simulink library "intertravamento"  (R2015a)
settings: Solver=ode45  SolverMode=SingleTasking  StartTime=0.0  StopTime=10.0  RelTol=1e-3
PostLoadFcn:
  | setsysloc_simulink(bdroot)
undefined symbols (not defined in the file or in its folder): docblock, getdatatypespecs, NumBits1, NumBits2, sfunxy, sigbuilder_block, slcm, SlDemoSign, Slope1, Slope2
libraries: simulink x46, sl_helperblocks x2, eml_lib x1
(part 5 of 6)

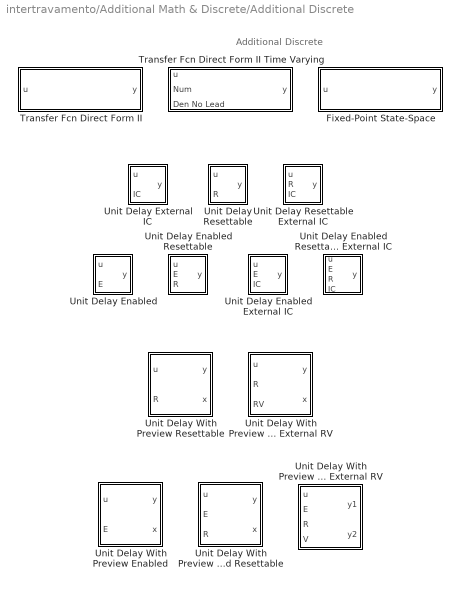
== system intertravamento/Additional Math & Discrete/Additional Discrete ==
  note: Additional Discrete
  Fixed-Point State-Space : Subsystem  mask(Fixed-Point State-Space){A=[2.6020 -2.2793 0.6708; 1 0 0; 0 1 0], B=[ 1; 0; 0], C=[0.0184    0.0024    0.0055], D=[0.0033], X0=0.0, InternalDataType=fixdt('double'), StateEqScaling=2^0, OutputEqScaling=2^0, LockScale=off, RndMeth=Floor, DoSatur=off}
      mask prompts: A "Simulink:masks:StateMatrixA_MP"; B "Simulink:masks:InputMatrixB_MP"; C "Simulink:masks:OutputMatrixC_MP"; D "Simulink:masks:DirectFeedthroughMatrixD_MP"; X0 "Simulink:masks:InitialConditionForState_MP"; InternalDataType "Simulink:masks:DataTypeForInternalCalculations_MP"; StateEqScaling "Simulink:masks:ScalingForStateEquationAXBU_MP"; OutputEqScaling "Simulink:masks:ScalingForOutputEquationCXDU_MP"; LockScale "Simulink:masks:LockOutputDataTypeAgainstFxpTools_MP"; RndMeth "Simulink:masks:IntegerRoundingMode_MP"; DoSatur "Simulink:masks:SaturateToMaxOrMinWhenOverflowsOccur_MP"
      mask help: Simulink:masks:FixedPointStateSpace_MD
      mask init:
      | blkH = gcbh;
      | blkName = getfullname(blkH);
      | 
      | vRndMeth = get_param(blkH,'RndMeth');
      | vDoSatur = get_param(blkH,'DoSatur');
      | blks = {'State Matrix A','Input Matrix B','Output Matrix C','Direct Link Matrix D','Sum Output Equation','Sum State Equation','Downcast Next State X','Downcast Output Y'};
      | for i = 1:length(blks)
      |   set_param([blkName,'/',blks{i}],'RndMeth',vRndMeth, ...
      | 	  'DoSatur',vDoSatur);
      | end
      mask TypeOptions RndMeth: Simulink:masks:Ceiling | Simulink:masks:Convergent | Simulink:masks:Floor | Simulink:masks:Nearest | Simulink:masks:Round | Simulink:masks:Simplest | Simulink:masks:Zero
      mask Display:
      | text(0.5, 0.5, 'y(n)=Cx(n)+Du(n)', 'horizontalAlignment', 'center', 'verticalAlignment', 'bottom');
      | text(0.5, 0.5, 'x(n+1)=Ax(n)+Bu(n)', 'horizontalAlignment', 'center', 'verticalAlignment', 'top');
  Transfer Fcn Direct Form II : Subsystem  mask(Transfer Fcn Direct Form II){NumCoefVec=[0.2 0.3 0.2], DenCoefVec=[-0.9    0.6], vinit=0.0, RndMeth=Floor, DoSatur=off}
      mask prompts: NumCoefVec "Simulink:masks:NumeratorCoefficients_MP"; DenCoefVec "Simulink:masks:DenominatorCoefficientsExcludingLead_MP"; vinit "Simulink:masks:InitialCondition_MP"; RndMeth "Simulink:masks:IntegerRoundingMode_MP"; DoSatur "Simulink:masks:SaturateToMaxOrMinWhenOverflowsOccur_MP"
      mask help: Simulink:masks:TransferFcnDirectFormII_MD
      mask init:
      | blkH = gcbh;
      | blkName = getfullname(blkH);
      | 
      | vRndMeth = get_param(blkH,'RndMeth');
      | vDoSatur = get_param(blkH,'DoSatur');
      | DCGain = polyval(NumCoefVec,1)./polyval([1 DenCoefVec],1);
      | maxGain = max( 1, max(max(abs(DCGain))) );
      | maxGain = max( maxGain, abs(NumCoefVec(1)) );
      | OutputSlopeMult = double(2^ceil(log2(maxGain)));
      | DCGain = (1)./polyval([1 DenCoefVec],1);
      | maxGain = max( 1, max(max(abs(DCGain))) );
      | OutputSlopeMult2 = double(2^ceil(log2(maxGain)));
      | set_param([blkName,'/NumCoef'],'RndMeth',vRndMeth, ...
      | 	'DoSatur',vDoSatur);
      | set_param([blkName,'/DenCoef'],'RndMeth',vRndMeth, ...
      | 	'DoSatur',vDoSatur);
      | set_param([blkName,'/Downcast'],'RndMeth',vRndMeth, ...
      | 	'DoSatur',vDoSatur);
      | set_param([blkName,'/Downcast1'],'RndMeth',vRndMeth, ...
      | 	'DoSatur',vDoSatur);
      | set_param([blkName,'/Sum'],'RndMeth',vRndMeth, ...
      | 	'DoSatur',vDoSatur);
      mask TypeOptions RndMeth: Simulink:masks:Ceiling | Simulink:masks:Convergent | Simulink:masks:Floor | Simulink:masks:Nearest | Simulink:masks:Round | Simulink:masks:Simplest | Simulink:masks:Zero
      mask Display: dpoly(NumCoefVec,[1 DenCoefVec],'z-')
  Transfer Fcn Direct Form II Time Varying : Subsystem  mask(Transfer Fcn Direct Form II Time Varying){vinit=0.0, RndMeth=Floor, DoSatur=off}
      mask prompts: vinit "Simulink:masks:InitialCondition_MP"; RndMeth "Simulink:masks:IntegerRoundingMode_MP"; DoSatur "Simulink:masks:SaturateToMaxOrMinWhenOverflowsOccur_MP"
      mask help: Simulink:masks:TransferFcnDirectFormIITimeVarying_MD
      mask init:
      | blkH = gcbh;
      | blkName = getfullname(blkH);
      | 
      | vRndMeth = get_param(blkH,'RndMeth');
      | vDoSatur = get_param(blkH,'DoSatur');
      | set_param([blkName,'/Dot1'],'RndMeth',vRndMeth, ...
      | 	'DoSatur',vDoSatur);
      | set_param([blkName,'/Dot2'],'RndMeth',vRndMeth, ...
      | 	'DoSatur',vDoSatur);
      | set_param([blkName,'/Downcast'],'RndMeth',vRndMeth, ...
      | 	'DoSatur',vDoSatur);
      | set_param([blkName,'/Downcast1'],'RndMeth',vRndMeth, ...
      | 	'DoSatur',vDoSatur);
      | set_param([blkName,'/Sum'],'RndMeth',vRndMeth, ...
      | 	'DoSatur',vDoSatur);
      mask TypeOptions RndMeth: Simulink:masks:Ceiling | Simulink:masks:Convergent | Simulink:masks:Floor | Simulink:masks:Nearest | Simulink:masks:Round | Simulink:masks:Simplest | Simulink:masks:Zero
      mask Display: fprintf('Direct\nForm II')
  Unit Delay Enabled : Subsystem  mask(Unit Delay Enabled){vinit=0.0, tsamp=-1}
      mask prompts: vinit "Simulink:masks:InitialCondition_MP"; tsamp "Simulink:masks:SampleTime_MP"
      mask help: Simulink:masks:UnitDelayEnabled_MD
      mask Display: dpoly(1,[1 0],'z')
  Unit Delay Enabled External IC : Subsystem  mask(Unit Delay Enabled External Initial Condition){tsamp=-1}
      mask prompts: tsamp "Simulink:masks:SampleTime_MP"
      mask help: Simulink:masks:UnitDelayEnabledExternalInitialCondition_MD
      mask Display: dpoly(1,[1 0],'z')
  Unit Delay Enabled Resettable : Subsystem  mask(Unit Delay Enabled Resettable){vinit=0.0, tsamp=-1}
      mask prompts: vinit "Simulink:masks:InitialCondition_MP"; tsamp "Simulink:masks:SampleTime_MP"
      mask help: Simulink:masks:UnitDelayEnabledResettable_MD
      mask Display: dpoly(1,[1 0],'z')
  Unit Delay Enabled Resettable External IC : Subsystem  mask(Unit Delay Enabled Resettable External Initial Condition){tsamp=-1}
      mask prompts: tsamp "Simulink:masks:SampleTime_MP"
      mask help: Simulink:masks:UnitDelayEnabledResettableExternalInitialCondition_MD
      mask Display: dpoly(1,[1 0],'z')
  Unit Delay External IC : Subsystem  mask(Unit Delay External Initial Condition){tsamp=-1}
      mask prompts: tsamp "Simulink:masks:SampleTime_MP"
      mask help: Simulink:masks:UnitDelayExternalInitialCondition_MD
      mask Display: dpoly(1,[1 0],'z')
  Unit Delay Resettable : Subsystem  mask(Unit Delay Resettable){vinit=0.0, tsamp=-1}
      mask prompts: vinit "Simulink:masks:InitialCondition_MP"; tsamp "Simulink:masks:SampleTime_MP"
      mask help: Simulink:masks:UnitDelayResettable_MD
      mask Display: dpoly(1,[1 0],'z')
  Unit Delay Resettable External IC : Subsystem  mask(Unit Delay Resettable External Initial Condition){tsamp=-1}
      mask prompts: tsamp "Simulink:masks:SampleTime_MP"
      mask help: Simulink:masks:UnitDelayResettableExternalInitialCondition_MD
      mask Display: dpoly(1,[1 0],'z')
  Unit Delay With Preview Enabled : Subsystem  mask(Unit Delay With Preview Enabled){vinit=0.0, tsamp=-1}
      mask prompts: vinit "Simulink:masks:InitialCondition_MP"; tsamp "Simulink:masks:SampleTime_MP"
      mask help: Simulink:masks:UnitDelayWithPreviewEnabled_MD
      mask Display:
      | plot([NaN 0.1 0.13 0.1 NaN 0.1 0.13 0.1 NaN 0.1 0.13 0.1 NaN -0.05 0.025 0.075 0.13 NaN -0.05 0.025 0.075 0.13 NaN 0.13 0.13 0.4475 0.4475 0.13 NaN 0.4475 0.4975 0.5525 0.5225 0.5525 0.5225 NaN 0.4475 0.4975 1.05 NaN 0.5525 0.5525 0.87 0.87 0.5525 NaN 0.71125 0.71125 NaN 0.6525 0.77 NaN 0.6525 0.77 0.6525 0.77 NaN 0.87 0.92 1.05 NaN 0.92 0.92 0.075 0.075 0.13],[NaN 0.846666666666667 0.816666666666667 0.786666666666667 NaN 0.58 0.55 0.52 NaN 0.313333333333333 0.283333333333333 0.253333333333333 NaN 0.75 0.75 0.816666666666667 0.816666666666667 NaN 0.25 0.25 0.55 0.55 NaN 0.15 0.95 0.95 0.15 0.15 NaN 0.55 0.35 0.35 0.38 0.35 0.32 NaN 0.55 0.75 0.75 NaN 0.15 0.55 0.55 0.15 0.15 NaN 0.5 0.4 NaN 0.35 0.35 NaN 0.3 0.3 0.2 0.2 NaN 0.35 0.25 0.25 NaN 0.25 0.05 0.05 0.283333333333333 0.283333333333333]);
      | text(0.23,0.806666666666667,'u');
      | text(0.23,0.54,'E');
  Unit Delay With Preview Enabled Resettable : Subsystem  mask(Unit Delay With Preview Enabled Resettable){vinit=0.0, tsamp=-1}
      mask prompts: vinit "Simulink:masks:InitialCondition_MP"; tsamp "Simulink:masks:SampleTime_MP"
      mask help: Simulink:masks:UnitDelayWithPreviewEnabledResettable_MD
      mask Display:
      | plot([NaN 0.1 0.13 0.1 NaN 0.1 0.13 0.1 NaN 0.1 0.13 0.1 NaN 0.1 0.13 0.1 NaN -0.05 0.025 0.075 0.13 NaN -0.05 0.025 0.075 0.13 NaN -0.05 0.025 0.075 0.13 NaN 0.13 0.13 0.4475 0.4475 0.13 NaN 0.4475 0.4975 0.5525 0.5225 0.5525 0.5225 NaN 0.4475 0.4975 1.05 NaN 0.5525 0.5525 0.87 0.87 0.5525 NaN 0.71125 0.71125 NaN 0.6525 0.77 NaN 0.6525 0.77 0.6525 0.77 NaN 0.87 0.92 1.05 NaN 0.92 0.92 0.075 0.075 0.13],[NaN 0.88 0.85 0.82 NaN 0.68 0.65 0.62 NaN 0.48 0.45 0.42 NaN 0.28 0.25 0.22 NaN 0.833333333333333 0.833333333333333 0.85 0.85 NaN 0.5 0.5 0.65 0.65 NaN 0.166666666666667 0.166666666666667 0.45 0.45 NaN 0.15 0.95 0.95 0.15 0.15 NaN 0.55 0.35 0.35 0.38 0.35 0.32 NaN 0.55 0.75 0.75 NaN 0.15 0.55 0.55 0.15 0.15 NaN 0.5 0.4 NaN 0.35 0.35 NaN 0.3 0.3 0.2 0.2 NaN 0.35 0.25 0.25 NaN 0.25 0.05 0.05 0.25 0.25]);
      | text(0.23,0.84,'u');
      | text(0.23,0.64,'E');
      | text(0.23,0.44,'R');
  Unit Delay With Preview Enabled Resettable External RV : Subsystem  mask(Unit Delay With Preview Enabled Resettable External RV){vinit=0.0, tsamp=-1}
      mask prompts: vinit "Simulink:masks:InitialCondition_MP"; tsamp "Simulink:masks:SampleTime_MP"
      mask help: Simulink:masks:UnitDelayWithPreviewEnabledResettableExternalRV_MD
      mask Display:
      | plot([NaN 0.1 0.13 0.1 NaN 0.1 0.13 0.1 NaN 0.1 0.13 0.1 NaN 0.1 0.13 0.1 NaN 0.1 0.13 0.1 NaN -0.05 0.025 0.075 0.13 NaN -0.05 0.025 0.075 0.13 NaN -0.05 0.025 0.075 0.13 NaN -0.05 0.025 0.075 0.13 NaN 0.13 0.13 0.4475 0.4475 0.13 NaN 0.4475 0.4975 0.5525 0.5225 0.5525 0.5225 NaN 0.4475 0.4975 1.05 NaN 0.5525 0.5525 0.87 0.87 0.5525 NaN 0.71125 0.71125 NaN 0.6525 0.77 NaN 0.6525 0.77 0.6525 0.77 NaN 0.87 0.92 1.05 NaN 0.92 0.92 0.075 0.075 0.13],[NaN 0.9 0.87 0.84 NaN 0.74 0.71 0.68 NaN 0.58 0.55 0.52 NaN 0.42 0.39 0.36 NaN 0.26 0.23 0.2 NaN 0.875 0.875 0.87 0.87 NaN 0.625 0.625 0.71 0.71 NaN 0.375 0.375 0.55 0.55 NaN 0.125 0.125 0.39 0.39 NaN 0.15 0.95 0.95 0.15 0.15 NaN 0.55 0.35 0.35 0.38 0.35 0.32 NaN 0.55 0.75 0.75 NaN 0.15 0.55 0.55 0.15 0.15 NaN 0.5 0.4 NaN 0.35 0.35 NaN 0.3 0.3 0.2 0.2 NaN 0.35 0.25 0.25 NaN 0.25 0.05 0.05 0.23 0.23]);
      | text(0.23,0.86,'u');
      | text(0.23,0.7,'E');
      | text(0.23,0.54,'R');
      | text(0.23,0.38,'RV');
  Unit Delay With Preview Resettable : Subsystem  mask(Unit Delay With Preview Resettable){vinit=0.0, tsamp=-1}
      mask prompts: vinit "Simulink:masks:InitialCondition_MP"; tsamp "Simulink:masks:SampleTime_MP"
      mask help: Simulink:masks:UnitDelayWithPreviewResettable_MD
      mask Display:
      | plot([NaN 0.1 0.13 0.1 NaN 0.1 0.13 0.1 NaN -0.05 0.025 0.075 0.13 NaN -0.05 0.025 0.075 0.13 NaN 0.13 0.13 0.4475 0.4475 0.13 NaN 0.4475 0.4975 0.5525 0.5225 0.5525 0.5225 NaN 0.4475 0.4975 1.05 NaN 0.5525 0.5525 0.87 0.87 0.5525 NaN 0.71125 0.71125 NaN 0.6525 0.77 NaN 0.6525 0.77 0.6525 0.77 NaN 0.87 0.92 1.05],[NaN 0.755 0.725 0.695 NaN 0.305 0.275 0.245 NaN 0.75 0.75 0.725 0.725 NaN 0.25 0.25 0.275 0.275 NaN 0.0499999999999999 0.95 0.95 0.0499999999999999 0.0499999999999999 NaN 0.5 0.275 0.275 0.305 0.275 0.245 NaN 0.5 0.75 0.75 NaN 0.0499999999999999 0.5 0.5 0.0499999999999999 0.0499999999999999 NaN 0.45 0.325 NaN 0.275 0.275 NaN 0.225 0.225 0.0999999999999999 0.0999999999999999 NaN 0.275 0.25 0.25]);
      | text(0.23,0.715,'u');
      | text(0.23,0.265,'R');
  Unit Delay With Preview Resettable External RV : Subsystem  mask(Unit Delay With Preview Resettable External RV){vinit=0.0, tsamp=-1}
      mask prompts: vinit "Simulink:masks:InitialCondition_MP"; tsamp "Simulink:masks:SampleTime_MP"
      mask help: Simulink:masks:UnitDelayWithPreviewResettableExternalRV_MD
      mask Display:
      | plot([NaN 0.1 0.13 0.1 NaN 0.1 0.13 0.1 NaN 0.1 0.13 0.1 NaN -0.05 0.025 0.075 0.13 NaN -0.05 0.025 0.075 0.13 NaN -0.05 0.025 0.075 0.13 NaN 0.13 0.13 0.4475 0.4475 0.13 NaN 0.4475 0.4975 0.5525 0.5225 0.5525 0.5225 NaN 0.4475 0.4975 1.05 NaN 0.5525 0.5525 0.87 0.87 0.5525 NaN 0.71125 0.71125 NaN 0.6525 0.77 NaN 0.6525 0.77 0.6525 0.77 NaN 0.87 0.92 1.05],[NaN 0.83 0.8 0.77 NaN 0.53 0.5 0.47 NaN 0.23 0.2 0.17 NaN 0.833333333333333 0.833333333333333 0.8 0.8 NaN 0.5 0.5 0.5 0.5 NaN 0.166666666666667 0.166666666666667 0.2 0.2 NaN 0.0499999999999999 0.95 0.95 0.0499999999999999 0.0499999999999999 NaN 0.5 0.275 0.275 0.305 0.275 0.245 NaN 0.5 0.75 0.75 NaN 0.0499999999999999 0.5 0.5 0.0499999999999999 0.0499999999999999 NaN 0.45 0.325 NaN 0.275 0.275 NaN 0.225 0.225 0.0999999999999999 0.0999999999999999 NaN 0.275 0.25 0.25]);
      | text(0.23,0.79,'u');
      | text(0.23,0.49,'R');
      | text(0.23,0.19,'RV');

== system intertravamento/Additional Math & Discrete/Additional Math: Increment - Decrement ==
  note: Increment/Decrement
  Decrement Real World : Subsystem  mask(Real World Value Decrement){}
      mask help: Simulink:masks:RealWorldValueDecrement_MD
      mask Display: disp('V--')
  Decrement Stored Integer : Subsystem  mask(Stored Integer Value Decrement){}
      mask help: Simulink:masks:StoredIntegerValueDecrement_MD
      mask Display: disp('Q--')
  Decrement To Zero : Subsystem  mask(Decrement To Zero){}
      mask help: Simulink:masks:DecrementToZero_MD
      mask Display: fprintf('max( V--, 0 )');
  Decrement Time To Zero : Subsystem  mask(Decrement Time To Zero){}
      mask help: Simulink:masks:DecrementTimeToZero_MD
      mask Display: fprintf('max( V-Ts, 0 )');
  Increment Real World : Subsystem  mask(Real World Value Increment){}
      mask help: Simulink:masks:RealWorldValueIncrement_MD
      mask Display: disp('V++')
  Increment Stored Integer : Subsystem  mask(Stored Integer Value Increment){}
      mask help: Simulink:masks:StoredIntegerValueIncrement_MD
      mask Display: disp('Q++')

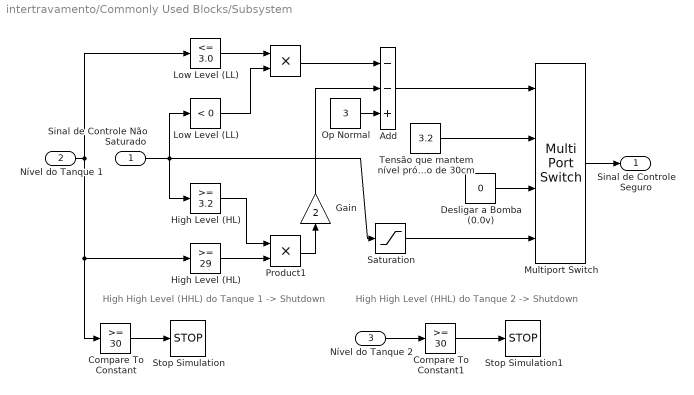
== system intertravamento/Commonly Used Blocks/Subsystem ==
  note: High High Level (HHL) do Tanque 2 -> Shutdown
  note: High High Level (HHL) do Tanque 1 -> Shutdown
  Sinal de Controle Não Saturado : Inport
  Nível do Tanque 1 : Inport  Port=2
  Nível do Tanque 2 : Inport  Port=3
  " " : Product
  " High Level (HL)" : simulink/Logic and Bit Operations/Compare To Constant  relop=>=  const=29  OutDataTypeStr=boolean
  " Low Level (LL) " : simulink/Logic and Bit Operations/Compare To Zero  relop=<  OutDataTypeStr=boolean
  Add : Sum  Inputs=--+
  Compare To Constant : simulink/Logic and Bit Operations/Compare To Constant  relop=>=  const=30  OutDataTypeStr=boolean
  Compare To Constant1 : simulink/Logic and Bit Operations/Compare To Constant  relop=>=  const=30  OutDataTypeStr=boolean
  Desligar a Bomba (0.0v) : Constant  Value=0
  Gain : Gain  Gain=2
  High Level (HL) : simulink/Logic and Bit Operations/Compare To Constant  relop=>=  const=3.2  OutDataTypeStr=boolean
  Low Level (LL) : simulink/Logic and Bit Operations/Compare To Constant  relop=<=  const=3.0  OutDataTypeStr=boolean
  Multiport Switch : MultiPortSwitch
  Op Normal : Constant  Value=3
  Product1 : Product
  Saturation : Saturate
  Stop Simulation : Stop
  Stop Simulation1 : Stop
  Tensão que mantem nível próximo de 30cm : Constant  Value=3.2
  Sinal de Controle Seguro : Outport
  wires:
  Multiport Switch/1 -> Sinal de Controle Seguro/1
  Sinal de Controle Não Saturado/1 -> " Low Level (LL) "/1, Saturation/1, High Level (HL)/1
  " High Level (HL)"/1 -> Product1/2
  High Level (HL)/1 -> Product1/1
  Low Level (LL)/1 -> " "/1
  " Low Level (LL) "/1 -> " "/2
  Saturation/1 -> Multiport Switch/4
  " "/1 -> Add/1
  Product1/1 -> Gain/1
  Gain/1 -> Add/2
  Op Normal/1 -> Add/3
  Add/1 -> Multiport Switch/1
  Tensão que mantem nível próximo de 30cm/1 -> Multiport Switch/2
  Desligar a Bomba (0.0v)/1 -> Multiport Switch/3
  Nível do Tanque 1/1 -> Compare To Constant/1, " High Level (HL)"/1, Low Level (LL)/1
  Compare To Constant/1 -> Stop Simulation/1
  Nível do Tanque 2/1 -> Compare To Constant1/1
  Compare To Constant1/1 -> Stop Simulation1/1

== system intertravamento/Continuous/PID Controller ==
  u : Inport  SampleTime=SampleTime
  Derivative Gain : Gain  DisableCoverage=on  Gain=D  ParamMin=DParamMin  ParamMax=DParamMax  OutMin=DOutMin  OutMax=DOutMax  SampleTime=SampleTime
  Filter : Integrator  DisableCoverage=on  InitialCondition=InitialConditionForFilter
  Filter Coefficient : Gain  Gain=N  ParamMin=NParamMin  ParamMax=NParamMax  OutMin=NOutMin  OutMax=NOutMax  SampleTime=SampleTime
  Integral Gain : Gain  DisableCoverage=on  Gain=I  ParamMin=IParamMin  ParamMax=IParamMax  OutMin=IOutMin  OutMax=IOutMax  SampleTime=SampleTime
  Integrator : Integrator  InitialCondition=InitialConditionForIntegrator
  Proportional Gain : Gain  Gain=P  ParamMin=PParamMin  ParamMax=PParamMax  OutMin=POutMin  OutMax=POutMax  SampleTime=SampleTime
  Sum : Sum  Inputs=+++  OutMin=SumOutMin  OutMax=SumOutMax  SampleTime=SampleTime
  SumD : Sum  DisableCoverage=on  Inputs=|+-  OutMin=SumDOutMin  OutMax=SumDOutMax  SampleTime=SampleTime
  y : Outport  SampleTime=SampleTime  InitialOutput=0
  wires:
  u/1 -> Proportional Gain/1, Integral Gain/1, Derivative Gain/1
  Proportional Gain/1 -> Sum/1
  Integral Gain/1 -> Integrator/1
  Derivative Gain/1 -> SumD/1
  SumD/1 -> Filter Coefficient/1
  Filter Coefficient/1 -> Filter/1, Sum/3
  Filter/1 -> SumD/2
  Integrator/1 -> Sum/2
  Sum/1 -> y/1

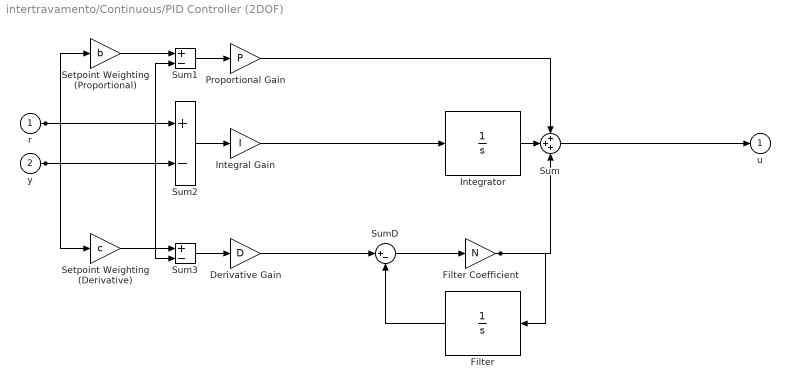
== system intertravamento/Continuous/PID Controller (2DOF) ==
  r : Inport  SampleTime=SampleTime
  y : Inport  Port=2  SampleTime=SampleTime
  Derivative Gain : Gain  DisableCoverage=on  Gain=D  ParamMin=DParamMin  ParamMax=DParamMax  OutMin=DOutMin  OutMax=DOutMax  SampleTime=SampleTime
  Filter : Integrator  DisableCoverage=on  InitialCondition=InitialConditionForFilter
  Filter Coefficient : Gain  Gain=N  ParamMin=NParamMin  ParamMax=NParamMax  OutMin=NOutMin  OutMax=NOutMax  SampleTime=SampleTime
  Integral Gain : Gain  DisableCoverage=on  Gain=I  ParamMin=IParamMin  ParamMax=IParamMax  OutMin=IOutMin  OutMax=IOutMax  SampleTime=SampleTime
  Integrator : Integrator  InitialCondition=InitialConditionForIntegrator
  Proportional Gain : Gain  Gain=P  ParamMin=PParamMin  ParamMax=PParamMax  OutMin=POutMin  OutMax=POutMax  SampleTime=SampleTime
  Setpoint Weighting (Derivative) : Gain  DisableCoverage=on  Gain=c  ParamMin=cParamMin  ParamMax=cParamMax  OutMin=cOutMin  OutMax=cOutMax  SampleTime=SampleTime
  Setpoint Weighting (Proportional) : Gain  DisableCoverage=on  Gain=b  ParamMin=bParamMin  ParamMax=bParamMax  OutMin=bOutMin  OutMax=bOutMax  SampleTime=SampleTime
  Sum : Sum  Inputs=+++  OutMin=SumOutMin  OutMax=SumOutMax  SampleTime=SampleTime
  Sum1 : Sum  DisableCoverage=on  Inputs=+-  OutMin=Sum1OutMin  OutMax=Sum1OutMax  SampleTime=SampleTime
  Sum2 : Sum  DisableCoverage=on  Inputs=+-  OutMin=Sum2OutMin  OutMax=Sum2OutMax  SampleTime=SampleTime
  Sum3 : Sum  DisableCoverage=on  Inputs=+-  OutMin=Sum3OutMin  OutMax=Sum3OutMax  SampleTime=SampleTime
  SumD : Sum  DisableCoverage=on  Inputs=|+-  OutMin=SumDOutMin  OutMax=SumDOutMax  SampleTime=SampleTime
  u : Outport  SampleTime=SampleTime  InitialOutput=0
  wires:
  r/1 -> Setpoint Weighting (Proportional)/1, Setpoint Weighting (Derivative)/1, Sum2/1
  y/1 -> Sum1/2, Sum2/2, Sum3/2
  Setpoint Weighting (Proportional)/1 -> Sum1/1
  Setpoint Weighting (Derivative)/1 -> Sum3/1
  Sum1/1 -> Proportional Gain/1
  Sum2/1 -> Integral Gain/1
  Sum3/1 -> Derivative Gain/1
  Proportional Gain/1 -> Sum/1
  Integral Gain/1 -> Integrator/1
  Derivative Gain/1 -> SumD/1
  SumD/1 -> Filter Coefficient/1
  Filter Coefficient/1 -> Filter/1, Sum/3
  Filter/1 -> SumD/2
  Integrator/1 -> Sum/2
  Sum/1 -> u/1

== system intertravamento/Discontinuities/Coulomb & Viscous Friction ==
  u : Inport
  Gain : Gain  DisableCoverage=on  Gain=gain  SaturateOnIntegerOverflow=on  OutDataTypeStr=Inherit: Same as input
  Gain1 : Gain  DisableCoverage=on  Gain=offset  OutDataTypeStr=Inherit: Inherit via back propagation  SaturateOnIntegerOverflow=on
  Sign : Signum  DisableCoverage=on
  Sum : Sum  Inputs=|++  SaturateOnIntegerOverflow=on  InputSameDT=on  OutDataTypeStr=Inherit: Same as first input
  y : Outport
  wires:
  Sign/1 -> Gain1/1
  u/1 -> Gain/1, Sign/1
  Gain1/1 -> Sum/1
  Sum/1 -> y/1
  Gain/1 -> Sum/2

== system intertravamento/Discontinuities/Dead Zone Dynamic ==
  up : Inport
  u : Inport  Port=2
  lo : Inport  Port=3
  Diff : Sum  Inputs=+-  InputSameDT=on  OutDataTypeStr=Inherit: Same as first input
  Switch : Switch  Criteria=u2 ~= 0  ZeroCross=off  InputSameDT=on
  Switch1 : Switch  Criteria=u2 ~= 0  ZeroCross=off  InputSameDT=on
  u_GTE_up : RelationalOperator  DisableCoverage=on  OutDataTypeStr=boolean  ZeroCross=off
  u_GT_lo : RelationalOperator  DisableCoverage=on  Operator=>  OutDataTypeStr=boolean  ZeroCross=off
  y : Outport
  wires:
  Switch1/1 -> Switch/3
  u/1 -> u_GT_lo/1, Switch1/1, u_GTE_up/1, Diff/1
  u_GT_lo/1 -> Switch1/2
  Diff/1 -> y/1
  Switch/1 -> Diff/2
  lo/1 -> u_GT_lo/2, Switch1/3
  u_GTE_up/1 -> Switch/2
  up/1 -> u_GTE_up/2, Switch/1

== system intertravamento/Discontinuities/Rate Limiter Dynamic ==
  note: U(k)
  note: Y(k)
  up : Inport
  u : Inport  Port=2
  lo : Inport  Port=3
  Delay Input2 : UnitDelay  Description=Store in Global RAM  DisableCoverage=on  SampleTime=-1
  Difference Inputs1 : Sum  Description=Add in CPU  DisableCoverage=on  Inputs=+-  OutDataTypeStr=Inherit: Inherit via back propagation
  Difference Inputs2 : Sum  Description=Add in CPU  OutDataTypeStr=Inherit: Inherit via back propagation
  FixPt Data Type Duplicate : DataTypeDuplicate  DisableCoverage=on  NumInputPorts=7
  Saturation Dynamic : simulink/Discontinuities/Saturation Dynamic  OutMin=[]  OutMax=[]  OutDataTypeStr=Inherit: Same as second input  OutDataType=fixdt(1, 16)  OutScaling=2^-10  DoSatur=off
  delta fall limit : Product  DisableCoverage=on  Inputs=**  OutDataTypeStr=Inherit: Inherit via back propagation  SaturateOnIntegerOverflow=on
  delta rise limit : Product  DisableCoverage=on  Inputs=**  OutDataTypeStr=Inherit: Inherit via back propagation  SaturateOnIntegerOverflow=on
  sample time : SampleTimeMath  DisableCoverage=on  TsampMathOp=Ts Only  weightValue=1
  Y : Outport  InitialOutput=0
  wires:
  sample time/1 -> delta rise limit/2, delta fall limit/2
  lo/1 -> delta fall limit/1
  delta rise limit/1 -> Saturation Dynamic/1, FixPt Data Type Duplicate/6
  up/1 -> delta rise limit/1
  Difference Inputs2/1 -> FixPt Data Type Duplicate/1, Delay Input2/1, Y/1
  Delay Input2/1 -> FixPt Data Type Duplicate/2, Difference Inputs1/2, Difference Inputs2/2  "Y(k-1)"
  Saturation Dynamic/1 -> FixPt Data Type Duplicate/7, Difference Inputs2/1
  delta fall limit/1 -> Saturation Dynamic/3, FixPt Data Type Duplicate/3
  u/1 -> sample time/1, FixPt Data Type Duplicate/5, Difference Inputs1/1
  Difference Inputs1/1 -> Saturation Dynamic/2, FixPt Data Type Duplicate/4  "( U(k) - Y(k-1) )"

== system intertravamento/Discontinuities/Saturation Dynamic ==
  up : Inport
  u : Inport  Port=2
  lo : Inport  Port=3
  Data Type Duplicate : DataTypeDuplicate  DisableCoverage=on
  Data Type Propagation : simulink/Signal Attributes/Data Type Propagation  PropDataType=fixdt(1, 16)  IfRefDouble=double  IfRefSingle=single  IsSigned=IsSigned1  NumBitsBase=NumBits1  NumBitsMult=1  NumBitsAdd=0  NumBitsAllowFinal=1:128  PropScaling=2^-10  ValuesUsedBestPrec=[5 -7]  SlopeBase=Slope1  SlopeMult=1  SlopeAdd=0  BiasBase=Bias1  BiasMult=1  BiasAdd=0
  LowerRelop1 : RelationalOperator  DisableCoverage=on  Operator=>  OutDataTypeStr=boolean
  Switch : Switch  Criteria=u2 ~= 0  OutDataTypeStr=Inherit: Inherit via back propagation  ZeroCross=off
  Switch2 : Switch  Criteria=u2 ~= 0  OutMin=OutMin  OutMax=OutMax  OutDataTypeStr=Inherit: Inherit via back propagation  ZeroCross=off
  UpperRelop : RelationalOperator  DisableCoverage=on  Operator=<  OutDataTypeStr=boolean
  y : Outport  OutMin=OutMin  OutMax=OutMax
  wires:
  UpperRelop/1 -> Switch/2
  LowerRelop1/1 -> Switch2/2
  Switch2/1 -> y/1, Data Type Duplicate/1
  Switch/1 -> Data Type Propagation/3, Switch2/3, Data Type Duplicate/2
  lo/1 -> UpperRelop/2, Switch/1
  u/1 -> UpperRelop/1, Switch/3, LowerRelop1/1, Data Type Propagation/1, Data Type Propagation/2
  up/1 -> LowerRelop1/2, Switch2/1

== system intertravamento/Discontinuities/Wrap To Zero ==
  note: U(k)
  U : Inport
  Constant : Constant  DisableCoverage=on  Value=0  OutDataTypeStr=Inherit: Inherit via back propagation
  FixPt Data Type Duplicate1 : DataTypeDuplicate  DisableCoverage=on  NumInputPorts=3
  FixPt Switch : Switch  Criteria=u2 > Threshold  Threshold=Threshold  OutDataTypeStr=Inherit: Inherit via back propagation  ZeroCross=off
  Y : Outport  InitialOutput=0
  wires:
  Constant/1 -> FixPt Data Type Duplicate1/3, FixPt Switch/1
  FixPt Switch/1 -> Y/1, FixPt Data Type Duplicate1/1
  U/1 -> FixPt Data Type Duplicate1/2, FixPt Switch/3, FixPt Switch/2

== system intertravamento/Discrete/Difference ==
  note: U(k)
  note: ( U(k) - U(k-1) )
  U : Inport
  Diff : Sum  Description=Add in CPU  Inputs=+-  OutMin=OutMin  OutMax=OutMax  OutDataTypeStr=OutDataTypeStr
  UD : UnitDelay  Description=Store in Global RAM  DisableCoverage=on  InitialCondition=ICPrevInput  SampleTime=-1
  Y : Outport  OutMin=OutMin  OutMax=OutMax  InitialOutput=0
  wires:
  U/1 -> UD/1, Diff/1
  UD/1 -> Diff/2  "U(k-1)"
  Diff/1 -> Y/1

== system intertravamento/Discrete/Discrete Derivative ==
  note: U(k)
  note: ( U(k) - U(k-1) )
  U : Inport
  Data Type Duplicate : DataTypeDuplicate  DisableCoverage=on  NumInputPorts=3
  Diff : Sum  Description=Add in CPU  Inputs=+-  OutMin=OutMin  OutMax=OutMax  OutDataTypeStr=diffDT
  TSamp : SampleTimeMath  DisableCoverage=on  TsampMathOp=/  weightValue=inverseGainval  TsampMathImp=Offline Scaling Adjustment
  UD : UnitDelay  Description=Store in Global RAM  DisableCoverage=on  InitialCondition=ICPrevScaledInput  SampleTime=-1
  Y : Outport  OutMin=OutMin  OutMax=OutMax  InitialOutput=0
  wires:
  TSamp/1 -> Data Type Duplicate/2, Diff/1, UD/1
  Diff/1 -> Data Type Duplicate/1, Y/1
  UD/1 -> Data Type Duplicate/3, Diff/2  "U(k-1)"
  U/1 -> TSamp/1

== system intertravamento/Discrete/First-Order Hold ==
  u : Inport  OutDataTypeStr=double
  Clock : Clock
      settings: DisableCoverage=on
  Digital Clock : DigitalClock  DisableCoverage=on  SampleTime=Ts
  Gain : Gain  DisableCoverage=on  Gain=1/Ts  SaturateOnIntegerOverflow=on  OutDataTypeStr=Inherit: Same as input  ParamDataTypeStr=Inherit: Same as input
  Hit Crossing : HitCross  DisableCoverage=on  HitCrossingOffset=1  HitCrossingDirection=rising  ShowOutputPort=off
  Output : Sum  Inputs=++|  SaturateOnIntegerOverflow=on  InputSameDT=on  OutDataTypeStr=Inherit: Same as first input
  Product : Product  DisableCoverage=on  SaturateOnIntegerOverflow=on  InputSameDT=on  OutDataTypeStr=Inherit: Same as first input
  Sum : Sum  DisableCoverage=on  Inputs=|+-  SaturateOnIntegerOverflow=on  InputSameDT=on  OutDataTypeStr=Inherit: Same as first input
  Sum2 : Sum  DisableCoverage=on  Inputs=|+-  SaturateOnIntegerOverflow=on  InputSameDT=on  OutDataTypeStr=Inherit: Same as first input
  Unit Delay : UnitDelay  DisableCoverage=on  SampleTime=Ts
  Zero-Order Hold : ZeroOrderHold  DisableCoverage=on  SampleTime=Ts
  y : Outport  OutDataTypeStr=double
  wires:
  Sum/1 -> Product/1
  Unit Delay/1 -> Sum/2
  Product/1 -> Output/2
  Zero-Order Hold/1 -> Output/1, Sum/1
  u/1 -> Zero-Order Hold/1, Unit Delay/1
  Clock/1 -> Sum2/1
  Digital Clock/1 -> Sum2/2
  Gain/1 -> Hit Crossing/1, Product/2
  Sum2/1 -> Gain/1
  Output/1 -> y/1

== system intertravamento/Discrete/Transfer Fcn First Order ==
  note: U(k)
  note: Y(k)
  U : Inport
  Data Type Duplicate : DataTypeDuplicate  DisableCoverage=on  NumInputPorts=3
  Diff : Sum  Description=Add in CPU  DisableCoverage=on  Inputs=+-
  Gain : Gain  DisableCoverage=on  Gain=PoleZ  OutDataTypeStr=Inherit: Inherit via back propagation
  Sum : Sum  Description=Add in CPU  OutDataTypeStr=Inherit: Inherit via back propagation
  UD : UnitDelay  Description=Store in Global RAM  DisableCoverage=on  InitialCondition=ICPrevOutput  SampleTime=-1
  Y : Outport  InitialOutput=0
  wires:
  Sum/1 -> Data Type Duplicate/1, UD/1, Y/1
  Gain/1 -> Data Type Duplicate/3, Sum/1  "(Pole) ( Y(k-1) - U(k) )"
  Diff/1 -> Gain/1  "( Y(k-1) - U(k) )"
  UD/1 -> Diff/1  "Y(k-1)"
  U/1 -> Data Type Duplicate/2, Sum/2, Diff/2

== system intertravamento/Discrete/Transfer Fcn Lead or Lag ==
  note: U(k)
  note: Y(k)
  u : Inport
  DataTypeProp : simulink/Signal Attributes/Data Type Propagation  PropDataType=fixdt(1, 16)  IfRefDouble=double  IfRefSingle=single  IsSigned=IsSigned1 or IsSigned2  NumBitsBase=max([NumBits1 NumBits2])  NumBitsMult=1  NumBitsAdd=0  NumBitsAllowFinal=1:128  PropScaling=2^-10  ValuesUsedBestPrec=[5 -7]  SlopeBase=min([Slope1 Slope2])  SlopeMult=OutputSlopeMult  SlopeAdd=0  BiasBase=Bias1  BiasMult=0  BiasAdd=0
  Delay Input : UnitDelay  Description=Store in Global RAM  DisableCoverage=on  InitialCondition=ICPrevInput  SampleTime=-1
      settings: AttributesFormatString=%<Description>
  Delay Output : UnitDelay  Description=Store in Global RAM  DisableCoverage=on  InitialCondition=ICPrevOutput  SampleTime=-1
      settings: AttributesFormatString=%<Description>
  Downcast : DataTypeConversion  Description=|  LockScale=on
      | Reduce from CPU Size
      |  to Global RAM Size
      settings: AttributesFormatString=%<Description>
  GainPole : Gain  Description=Multiply in CPU  DisableCoverage=on  Gain=PoleZ  LockScale=on
      settings: AttributesFormatString=%<Description>
  GainZero : Gain  Description=Multiply in CPU  DisableCoverage=on  Gain=ZeroZ  LockScale=on
      settings: AttributesFormatString=%<Description>
  Sum : Sum  Description=Add in CPU  DisableCoverage=on  Inputs=+-+  LockScale=on
      settings: AttributesFormatString=%<Description>
  y : Outport  InitialOutput=0
  wires:
  Downcast/1 -> DataTypeProp/3, Delay Output/1, y/1
  Sum/1 -> Downcast/1  "(Pole) Y(k-1) + U(k) - (Zero) U(k-1)"
  GainPole/1 -> Sum/3  "(Pole) Y(k-1)"
  GainZero/1 -> Sum/2  "(Zero) U(k-1)"
  Delay Input/1 -> GainZero/1  "U(k-1)"
  Delay Output/1 -> GainPole/1  "Y(k-1)"
  u/1 -> Delay Input/1, Sum/1, DataTypeProp/1, DataTypeProp/2

== system intertravamento/Discrete/Transfer Fcn Real Zero ==
  note: U(k)
  note: U(k) - (Zero) U(k-1)
  u : Inport
  DataTypeProp : simulink/Signal Attributes/Data Type Propagation  PropDataType=fixdt(1, 16)  IfRefDouble=double  IfRefSingle=single  IsSigned=IsSigned1 or IsSigned2  NumBitsBase=max([NumBits1 NumBits2])  NumBitsMult=1  NumBitsAdd=0  NumBitsAllowFinal=1:128  PropScaling=2^-10  ValuesUsedBestPrec=[5 -7]  SlopeBase=min([Slope1 Slope2])  SlopeMult=OutputSlopeMult  SlopeAdd=0  BiasBase=Bias1  BiasMult=0  BiasAdd=0
  Delay Input : UnitDelay  Description=Store in Global RAM  DisableCoverage=on  InitialCondition=ICPrevInput  SampleTime=-1
  GainZero : Gain  Description=Multiply in CPU  DisableCoverage=on  Gain=ZeroZ  LockScale=on
  Sum : Sum  Description=Add in CPU  Inputs=+-  OutDataTypeStr=Inherit: Inherit via back propagation  LockScale=on
  y : Outport  InitialOutput=0
  wires:
  u/1 -> DataTypeProp/2, DataTypeProp/1, Sum/1, Delay Input/1
  Delay Input/1 -> GainZero/1  "U(k-1)"
  GainZero/1 -> Sum/2  "(Zero) U(k-1)"
  Sum/1 -> y/1, DataTypeProp/3

== system intertravamento/Logic and Bit Operations/Bit Clear ==
  u : Inport
  FixPt Bitwise Operator3 : simulink/Logic and Bit Operations/Bitwise Operator  logicop=OR  UseBitMask=on  BitMask=2.^iBit  BitMaskRealWorld=Stored Integer
  FixPt Bitwise Operator4 : simulink/Logic and Bit Operations/Bitwise Operator  logicop=NOT  UseBitMask=off  BitMask=2^iBit  BitMaskRealWorld=Stored Integer
  FixPt Bitwise Operator5 : simulink/Logic and Bit Operations/Bitwise Operator  logicop=NOT  UseBitMask=off  BitMask=2^iBit  BitMaskRealWorld=Stored Integer
  y : Outport
  wires:
  FixPt Bitwise Operator3/1 -> FixPt Bitwise Operator5/1
  FixPt Bitwise Operator4/1 -> FixPt Bitwise Operator3/1
  u/1 -> FixPt Bitwise Operator4/1
  FixPt Bitwise Operator5/1 -> y/1

== system intertravamento/Logic and Bit Operations/Bit Set ==
  u : Inport
  FixPt Bitwise Operator1 : simulink/Logic and Bit Operations/Bitwise Operator  logicop=OR  UseBitMask=on  BitMask=2.^iBit  BitMaskRealWorld=Stored Integer
  y : Outport
  wires:
  FixPt Bitwise Operator1/1 -> y/1
  u/1 -> FixPt Bitwise Operator1/1

== system intertravamento/Logic and Bit Operations/Compare To Constant ==
  u : Inport
  Compare : RelationalOperator  Operator=<=  OutDataTypeStr=boolean  InputSameDT=on
  Constant : Constant  DisableCoverage=on  Value=const  OutDataTypeStr=Inherit: Inherit via back propagation
  y : Outport
  wires:
  Compare/1 -> y/1
  Constant/1 -> Compare/2
  u/1 -> Compare/1

== system intertravamento/Logic and Bit Operations/Compare To Zero ==
  u : Inport
  Compare : RelationalOperator  Operator=<=  OutDataTypeStr=boolean  InputSameDT=on
  Constant : Constant  DisableCoverage=on  Value=0  OutDataTypeStr=Inherit: Inherit via back propagation  PreserveConstantTs=on
  y : Outport
  wires:
  Compare/1 -> y/1
  u/1 -> Compare/1
  Constant/1 -> Compare/2

== system intertravamento/Logic and Bit Operations/Detect Change ==
  note: U(k)
  note: Edge
  U : Inport
  Delay Input1 : UnitDelay  Description=Store in Global RAM  DisableCoverage=on  InitialCondition=vinit  SampleTime=-1
  FixPt Relational Operator : RelationalOperator  Operator=~=  OutDataTypeStr=boolean  ZeroCross=off
  Y : Outport  InitialOutput=0
  wires:
  U/1 -> Delay Input1/1, FixPt Relational Operator/1
  Delay Input1/1 -> FixPt Relational Operator/2  "U(k-1)"
  FixPt Relational Operator/1 -> Y/1

== system intertravamento/Logic and Bit Operations/Detect Decrease ==
  note: U(k)
  note: Edge
  U : Inport
  Delay Input1 : UnitDelay  Description=Store in Global RAM  DisableCoverage=on  InitialCondition=vinit  SampleTime=-1
  FixPt Relational Operator : RelationalOperator  Operator=<  OutDataTypeStr=boolean  ZeroCross=off
  Y : Outport  InitialOutput=0
  wires:
  FixPt Relational Operator/1 -> Y/1
  Delay Input1/1 -> FixPt Relational Operator/2  "U(k-1)"
  U/1 -> FixPt Relational Operator/1, Delay Input1/1

== system intertravamento/Logic and Bit Operations/Detect Increase ==
  note: U(k)
  note: Edge
  U : Inport
  Delay Input1 : UnitDelay  Description=Store in Global RAM  DisableCoverage=on  InitialCondition=vinit  SampleTime=-1
  FixPt Relational Operator : RelationalOperator  Operator=>  OutDataTypeStr=boolean  ZeroCross=off
  Y : Outport  InitialOutput=0
  wires:
  U/1 -> Delay Input1/1, FixPt Relational Operator/1
  Delay Input1/1 -> FixPt Relational Operator/2  "U(k-1)"
  FixPt Relational Operator/1 -> Y/1

== system intertravamento/Logic and Bit Operations/Detect Fall Negative ==
  note: U(k)
  note: Edge
  U : Inport
  Delay Input1 : UnitDelay  Description=Store in Global RAM  DisableCoverage=on  InitialCondition=vinit  SampleTime=-1
  FixPt Relational Operator : RelationalOperator  Operator=>  OutDataTypeStr=boolean  ZeroCross=off
  Negative : simulink/Logic and Bit Operations/Compare To Zero  relop=<  OutDataTypeStr=uint8  ZeroCross=off
  Y : Outport  InitialOutput=0
  wires:
  Negative/1 -> FixPt Relational Operator/1, Delay Input1/1  "U(k)"
  FixPt Relational Operator/1 -> Y/1
  Delay Input1/1 -> FixPt Relational Operator/2  "U(k-1)"
  U/1 -> Negative/1

== system intertravamento/Logic and Bit Operations/Detect Fall Nonpositive ==
  note: U(k)
  note: Edge
  U : Inport
  Delay Input1 : UnitDelay  Description=Store in Global RAM  DisableCoverage=on  InitialCondition=vinit  SampleTime=-1
  FixPt Relational Operator : RelationalOperator  Operator=>  OutDataTypeStr=boolean  ZeroCross=off
  Nonpositive : simulink/Logic and Bit Operations/Compare To Zero  relop=<=  OutDataTypeStr=uint8  ZeroCross=off
  Y : Outport  InitialOutput=0
  wires:
  U/1 -> Nonpositive/1
  Delay Input1/1 -> FixPt Relational Operator/2  "U(k-1)"
  FixPt Relational Operator/1 -> Y/1
  Nonpositive/1 -> Delay Input1/1, FixPt Relational Operator/1  "U(k)"

== system intertravamento/Logic and Bit Operations/Detect Rise Nonnegative ==
  note: U(k)
  note: Edge
  U : Inport
  Delay Input1 : UnitDelay  Description=Store in Global RAM  DisableCoverage=on  InitialCondition=vinit  SampleTime=-1
  FixPt Relational Operator : RelationalOperator  Operator=>  OutDataTypeStr=boolean  ZeroCross=off
  Nonnegative : simulink/Logic and Bit Operations/Compare To Zero  relop=>=  OutDataTypeStr=uint8  ZeroCross=off
  Y : Outport  InitialOutput=0
  wires:
  U/1 -> Nonnegative/1
  Delay Input1/1 -> FixPt Relational Operator/2  "U(k-1)"
  FixPt Relational Operator/1 -> Y/1
  Nonnegative/1 -> Delay Input1/1, FixPt Relational Operator/1  "U(k)"

== system intertravamento/Logic and Bit Operations/Detect Rise Positive ==
  note: U(k)
  note: Edge
  U : Inport
  Delay Input1 : UnitDelay  Description=Store in Global RAM  DisableCoverage=on  InitialCondition=vinit  SampleTime=-1
  FixPt Relational Operator : RelationalOperator  Operator=>  OutDataTypeStr=boolean  ZeroCross=off
  Positive : simulink/Logic and Bit Operations/Compare To Zero  relop=>  OutDataTypeStr=uint8  ZeroCross=off
  Y : Outport  InitialOutput=0
  wires:
  Positive/1 -> FixPt Relational Operator/1, Delay Input1/1  "U(k)"
  FixPt Relational Operator/1 -> Y/1
  Delay Input1/1 -> FixPt Relational Operator/2  "U(k-1)"
  U/1 -> Positive/1

== system intertravamento/Logic and Bit Operations/Extract Bits ==
  u : Inport
  DTProp1 : simulink/Signal Attributes/Data Type Propagation  PropDataType=fixdt(1, 16)  IfRefDouble=double  IfRefSingle=single  IsSigned=IsSigned1  NumBitsBase=NumBits1  NumBitsMult=0.5  NumBitsAdd=0  NumBitsAllowFinal=1:128  PropScaling=2^-10  ValuesUsedBestPrec=[5 -7]  SlopeBase=PosRange1  SlopeMult=2^0  SlopeAdd=0  BiasBase=Bias1  BiasMult=1  BiasAdd=0
  DTProp2 : simulink/Signal Attributes/Data Type Propagation  PropDataType=fixdt(1, 16)  IfRefDouble=double  IfRefSingle=single  IsSigned=IsSigned1  NumBitsBase=NumBits1  NumBitsMult=1  NumBitsAdd=0  NumBitsAllowFinal=1:128  PropScaling=1  ValuesUsedBestPrec=[5 -7]  SlopeBase=Slope1  SlopeMult=1  SlopeAdd=0  BiasBase=Bias1  BiasMult=1  BiasAdd=0
  Extract Desired Bits : DataTypeConversion  DisableCoverage=on
  Modify Scaling Only : DataTypeConversion  ConvertRealWorld=Stored Integer (SI)
  y : Outport
  wires:
  Extract Desired Bits/1 -> DTProp1/3, Modify Scaling Only/1, DTProp2/2, DTProp2/1
  u/1 -> DTProp1/1, DTProp1/2, Extract Desired Bits/1
  Modify Scaling Only/1 -> y/1, DTProp2/3

== system intertravamento/Logic and Bit Operations/Interval Test ==
  u : Inport
  AND : Logic  AllPortsSameDT=off  OutDataTypeStr=boolean
  FixPt Data Type Duplicate : DataTypeDuplicate  DisableCoverage=on  NumInputPorts=3
  Lower Limit : Constant  DisableCoverage=on  Value=lowlimit  OutDataTypeStr=Inherit: Inherit via back propagation
  Lower Test : RelationalOperator  DisableCoverage=on  Operator=<=  OutDataTypeStr=boolean  ZeroCross=off
  Upper Limit : Constant  DisableCoverage=on  Value=uplimit  OutDataTypeStr=Inherit: Inherit via back propagation
  Upper Test : RelationalOperator  DisableCoverage=on  Operator=<=  OutDataTypeStr=boolean  ZeroCross=off
  y : Outport
  wires:
  Lower Limit/1 -> Lower Test/1, FixPt Data Type Duplicate/2
  Upper Limit/1 -> Upper Test/2, FixPt Data Type Duplicate/3
  Lower Test/1 -> AND/1
  Upper Test/1 -> AND/2
  u/1 -> FixPt Data Type Duplicate/1, Lower Test/2, Upper Test/1
  AND/1 -> y/1

== system intertravamento/Logic and Bit Operations/Interval Test Dynamic ==
  up : Inport
  u : Inport  Port=2
  lo : Inport  Port=3
  FixPt Data Type Duplicate : DataTypeDuplicate  DisableCoverage=on  NumInputPorts=3
  FixPt Logical Operator : Logic  AllPortsSameDT=off  OutDataTypeStr=boolean
  Lower Test : RelationalOperator  DisableCoverage=on  Operator=<=  OutDataTypeStr=boolean  ZeroCross=off
  Upper Test : RelationalOperator  DisableCoverage=on  Operator=<=  OutDataTypeStr=boolean  ZeroCross=off
  y : Outport
  wires:
  FixPt Logical Operator/1 -> y/1
  u/1 -> Lower Test/2, Upper Test/1, FixPt Data Type Duplicate/2
  Upper Test/1 -> FixPt Logical Operator/2
  Lower Test/1 -> FixPt Logical Operator/1
  up/1 -> Upper Test/2, FixPt Data Type Duplicate/3
  lo/1 -> Lower Test/1, FixPt Data Type Duplicate/1

== system intertravamento/Lookup Tables/Cosine ==
  u : Inport
  Cosine : sl_helperblocks/Cosine  NumDataPoints=NumDataPoints  OutputWordLength=OutputWordLength  InternalRulePriority=Precision
  cos(2*pi*u) : Outport
  wires:
  Cosine/1 -> cos(2*pi*u)/1
  u/1 -> Cosine/1

== system intertravamento/Lookup Tables/Sine ==
  u : Inport
  Sine : sl_helperblocks/Sine  NumDataPoints=NumDataPoints  OutputWordLength=OutputWordLength  InternalRulePriority=Precision
  sin(2*pi*u) : Outport
  wires:
  Sine/1 -> sin(2*pi*u)/1
  u/1 -> Sine/1

== system intertravamento/Math Operations/Algebraic Constraint ==
  f(z) : Inport
  Initial Guess : InitialCondition  Value=z0
  Sum : Sum  DisableCoverage=on  Inputs=|++  SaturateOnIntegerOverflow=on  InputSameDT=on  OutDataTypeStr=Inherit: Same as first input
  z : Outport
  wires:
  f(z)/1 -> Sum/1
  Initial Guess/1 -> z/1, Sum/2
  Sum/1 -> Initial Guess/1

== system intertravamento/Math Operations/MinMax Running Resettable ==
  note: Reset
  u : Inport
  R : Inport  Port=2
  Data Type Duplicate : DataTypeDuplicate  DisableCoverage=on  NumInputPorts=3
  MinMax : MinMax  DisableCoverage=on  Inputs=2  OutDataTypeStr=Inherit: Inherit via back propagation  ZeroCross=off
      settings: LockScale=on
  Unit Delay With Preview Resettable : simulink/Additional Math & Discrete/Additional Discrete/Unit Delay With Preview Resettable  vinit=vinit  tsamp=-1
  y : Outport
  wires:
  Unit Delay With Preview Resettable/1 -> y/1
  MinMax/1 -> Data Type Duplicate/1, Unit Delay With Preview Resettable/1
  Unit Delay With Preview Resettable/2 -> Data Type Duplicate/2, MinMax/2
  u/1 -> Data Type Duplicate/3, MinMax/1
  R/1 -> Unit Delay With Preview Resettable/2

== system intertravamento/Math Operations/Slider Gain ==
  u : Inport
  Slider Gain : Gain  Gain=gain  SaturateOnIntegerOverflow=on  OutDataTypeStr=Inherit: Same as input  ParamDataTypeStr=Inherit: Same as input
  y : Outport
  wires:
  Slider Gain/1 -> y/1
  u/1 -> Slider Gain/1

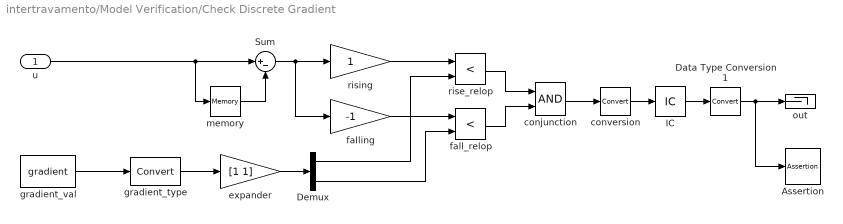
== system intertravamento/Model Verification/Check Discrete Gradient ==
  u : Inport
  Assertion : Assertion  DisableCoverage=on  AssertionFailFcn=evalin('base',callback)
  Data Type Conversion1 : DataTypeConversion  DisableCoverage=on  SaturateOnIntegerOverflow=on  RndMeth=Zero
  Demux : Demux  DisableCoverage=on  Outputs=2
  IC : InitialCondition  DisableCoverage=on
  Sum : Sum  DisableCoverage=on  Inputs=|+-  SaturateOnIntegerOverflow=on  InputSameDT=on  OutDataTypeStr=Inherit: Same as first input
  conjunction : Logic  DisableCoverage=on
  conversion : DataTypeConversion  DisableCoverage=on  SaturateOnIntegerOverflow=on  RndMeth=Zero
  expander : Gain  DisableCoverage=on  Gain=[1 1]  SaturateOnIntegerOverflow=on  OutDataTypeStr=Inherit: Same as input  ParamDataTypeStr=Inherit: Same as input
  fall_relop : RelationalOperator  DisableCoverage=on  Operator=<  InputSameDT=on
  falling : Gain  DisableCoverage=on  Gain=-1  SaturateOnIntegerOverflow=on  OutDataTypeStr=Inherit: Same as input  ParamDataTypeStr=Inherit: Same as input
  gradient_type : DataTypeConversion  DisableCoverage=on  SaturateOnIntegerOverflow=on  RndMeth=Zero
  gradient_val : Constant  DisableCoverage=on  Value=gradient
  memory : Memory  DisableCoverage=on  InheritSampleTime=on
  out : Terminator
  rise_relop : RelationalOperator  DisableCoverage=on  Operator=<  InputSameDT=on
  rising : Gain  DisableCoverage=on  SaturateOnIntegerOverflow=on  OutDataTypeStr=Inherit: Same as input  ParamDataTypeStr=Inherit: Same as input
  wires:
  Data Type Conversion1/1 -> Assertion/1, out/1
  conversion/1 -> IC/1
  IC/1 -> Data Type Conversion1/1
  conjunction/1 -> conversion/1
  fall_relop/1 -> conjunction/2
  rise_relop/1 -> conjunction/1
  falling/1 -> fall_relop/1
  rising/1 -> rise_relop/1
  Sum/1 -> rising/1, falling/1
  memory/1 -> Sum/2
  Demux/2 -> fall_relop/2
  Demux/1 -> rise_relop/2
  expander/1 -> Demux/1
  u/1 -> Sum/1, memory/1
  gradient_val/1 -> gradient_type/1
  gradient_type/1 -> expander/1

== system intertravamento/Model Verification/Check Dynamic Gap ==
  max : Inport
  min : Inport  Port=2
  u : Inport  Port=3
  Assertion : Assertion  DisableCoverage=on  AssertionFailFcn=evalin('base',callback)
  disjunction : Logic  DisableCoverage=on  Operator=OR
  max_relop : RelationalOperator  DisableCoverage=on  Operator=<
  min_relop : RelationalOperator  DisableCoverage=on  Operator=<
  out : Terminator
  wires:
  max/1 -> max_relop/1
  min/1 -> min_relop/2
  u/1 -> min_relop/1, max_relop/2
  disjunction/1 -> Assertion/1, out/1
  min_relop/1 -> disjunction/2
  max_relop/1 -> disjunction/1

== system intertravamento/Model Verification/Check Dynamic Range ==
  max : Inport
  min : Inport  Port=2
  u : Inport  Port=3
  Assertion : Assertion  DisableCoverage=on  AssertionFailFcn=evalin('base',callback)
  conjunction : Logic  DisableCoverage=on
  max_relop : RelationalOperator  DisableCoverage=on  Operator=<
  min_relop : RelationalOperator  DisableCoverage=on  Operator=<
  out : Terminator
  wires:
  u/1 -> max_relop/1, min_relop/2
  min/1 -> min_relop/1
  max/1 -> max_relop/2
  min_relop/1 -> conjunction/1
  max_relop/1 -> conjunction/2
  conjunction/1 -> Assertion/1, out/1

== system intertravamento/Model Verification/Check Static Gap ==
  u : Inport
  Assertion : Assertion  DisableCoverage=on  AssertionFailFcn=evalin('base',callback)
  disjunction : Logic  DisableCoverage=on  Operator=OR
  max_relop : RelationalOperator  DisableCoverage=on  Operator=<=
  max_val : Constant  DisableCoverage=on  Value=max
  min_relop : RelationalOperator  DisableCoverage=on  Operator=<=
  min_val : Constant  DisableCoverage=on  Value=min
  out : Terminator
  wires:
  min_val/1 -> min_relop/2
  max_val/1 -> max_relop/1
  u/1 -> max_relop/2, min_relop/1
  max_relop/1 -> disjunction/1
  min_relop/1 -> disjunction/2
  disjunction/1 -> Assertion/1, out/1

== system intertravamento/Model Verification/Check Static Range ==
  u : Inport
  Assertion : Assertion  DisableCoverage=on  AssertionFailFcn=evalin('base',callback)
  conjunction : Logic  DisableCoverage=on
  max_relop : RelationalOperator  DisableCoverage=on  Operator=<=
  max_val : Constant  DisableCoverage=on  Value=max
  min_relop : RelationalOperator  DisableCoverage=on  Operator=<=
  min_val : Constant  DisableCoverage=on  Value=min
  out : Terminator
  wires:
  conjunction/1 -> Assertion/1, out/1
  max_relop/1 -> conjunction/2
  min_relop/1 -> conjunction/1
  max_val/1 -> max_relop/2
  min_val/1 -> min_relop/1
  u/1 -> max_relop/1, min_relop/2

== system intertravamento/Model Verification/Check Dynamic Lower Bound ==
  min : Inport  DisableCoverage=on
  u : Inport  Port=2
  Assertion : Assertion  DisableCoverage=on  AssertionFailFcn=evalin('base',callback)
  min_relop : RelationalOperator  DisableCoverage=on  Operator=<
  out : Terminator
  wires:
  u/1 -> min_relop/2
  min/1 -> min_relop/1
  min_relop/1 -> Assertion/1, out/1

== system intertravamento/Model Verification/Check Dynamic Upper Bound ==
  max : Inport
  u : Inport  Port=2
  Assertion : Assertion  DisableCoverage=on  AssertionFailFcn=evalin('base',callback)
  max_relop : RelationalOperator  DisableCoverage=on  Operator=<
  out : Terminator
  wires:
  u/1 -> max_relop/1
  max/1 -> max_relop/2
  max_relop/1 -> Assertion/1, out/1

== system intertravamento/Model Verification/Check Input Resolution ==
  u : Inport
  Assertion : Assertion  DisableCoverage=on  AssertionFailFcn=evalin('base',callback)
  dead_out : Terminator
  dead_resolution : Constant  DisableCoverage=on  Value=[1 1]
  dead_u : Constant  DisableCoverage=on
  fixed : Subsystem  DisableCoverage=on
  out : Terminator
  resolution : Constant  DisableCoverage=on  Value=resolution
  resolution_type : DataTypeConversion  DisableCoverage=on  SaturateOnIntegerOverflow=on  RndMeth=Zero
  steps : Subsystem  DisableCoverage=on
  wires:
  resolution/1 -> resolution_type/1
  u/1 -> steps/1(u)
  resolution_type/1 -> steps/2(resolution)
  steps/1(out) -> Assertion/1, out/1
  dead_u/1 -> fixed/1(u)
  dead_resolution/1 -> fixed/2(resolution)
  fixed/1(out) -> dead_out/1

== system intertravamento/Model Verification/Check Static Lower Bound ==
  u : Inport
  Assertion : Assertion  DisableCoverage=on  AssertionFailFcn=evalin('base',callback)
  min_relop : RelationalOperator  DisableCoverage=on  Operator=<=
  min_val : Constant  DisableCoverage=on  Value=min
  out : Terminator
  wires:
  min_relop/1 -> Assertion/1, out/1
  u/1 -> min_relop/2
  min_val/1 -> min_relop/1

== system intertravamento/Model Verification/Check Static Upper Bound ==
  u : Inport
  Assertion : Assertion  DisableCoverage=on  AssertionFailFcn=evalin('base',callback)
  max_relop : RelationalOperator  DisableCoverage=on  Operator=<=
  max_val : Constant  DisableCoverage=on  Value=max
  out : Terminator
  wires:
  u/1 -> max_relop/1
  max_val/1 -> max_relop/2
  max_relop/1 -> Assertion/1, out/1
